simulink model "MAXWELL_Simulink"  (R2023a)
settings: Solver=FixedStepAuto  StartTime=0.0  StopTime=3600*4  FixedStep=5  MaxStep=10  RelTol=1e-7  AbsTol=1e-7
model workspace (MAT data in the model file):
  Gs = [0  0  0.707106781187  -0.707106781187; 0.707106781187  0.707106781187  -0.707106781187  -0.707106781187; 0.707106781187  -0.707106781187  0  0]
  Iws = 0.002
  OmegaRW_0 = [5000; 5000; 5000; 5000]
  Omega_bias = 26.1799
  RW_bias = 52.3598775598
undefined symbols (not defined in the file or in its folder): DiscIntNeverNeededParam, rad, s
libraries: slpidlib x3, dspinverses x3, sharedtransform x3, aerolibconvert2 x1, aerolibsatdyn x1, dspmathops x1, aerolibutil x1
settings Model: Creator=The MathWorks, Inc.  LastModifiedBy=TheBa
settings SolverCC: MaxConsecutiveMinStep=10  AutoInsertRateTranBlk=on  DecoupledContinuousIntegration=on  MinimalZcImpactIntegration=on  MaxZcPerStep=1
settings OptimizationCC: DefaultParameterBehavior=Inlined  UseDivisionForNetSlopeComputation=on  GainParamInheritBuiltInType=on  UseFloatMulNetSlope=on  InlineInvariantSignals=on  EfficientFloat2IntCast=on  LifeSpan=1
settings DebuggingCC: ReadBeforeWriteMsg=DisableAll  WriteAfterWriteMsg=DisableAll  WriteAfterReadMsg=DisableAll  MultiTaskDSMMsg=none  UnconnectedInputMsg=warning  UnconnectedOutputMsg=warning  UnconnectedLineMsg=warning
settings HardwareCC: ProdLongLongMode=on
settings ModelReferenceCC: UpdateModelReferenceTargets=IfOutOfDate  EnableRefExpFcnMdlSchedulingChecks=on
settings SFSimCC: SFSimEcho=off  MATLABDynamicMemAlloc=off
settings RTWCC: GenerateReport=on  BuildConfiguration=Faster Runs  LaunchReport=on  DLArmComputeVersion=19.05
settings CodeAppCC: ForceParamTrailComments=on
settings GRTTargetCC: CombineSignalStateStructs=on  MatFileLogging=off  SupportNonFinite=off  SupportVariableSizeSignals=on

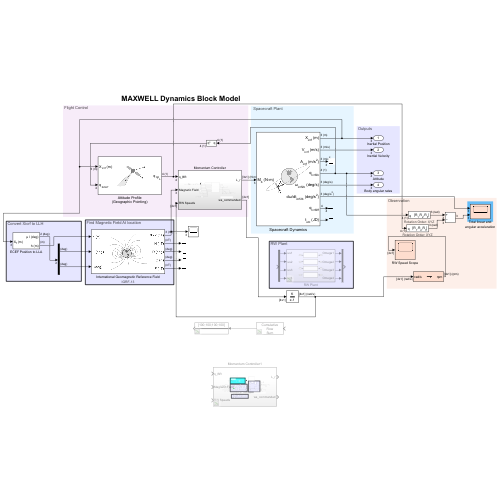
[thumbnail: Simulink's stored preview of the top-level diagram]
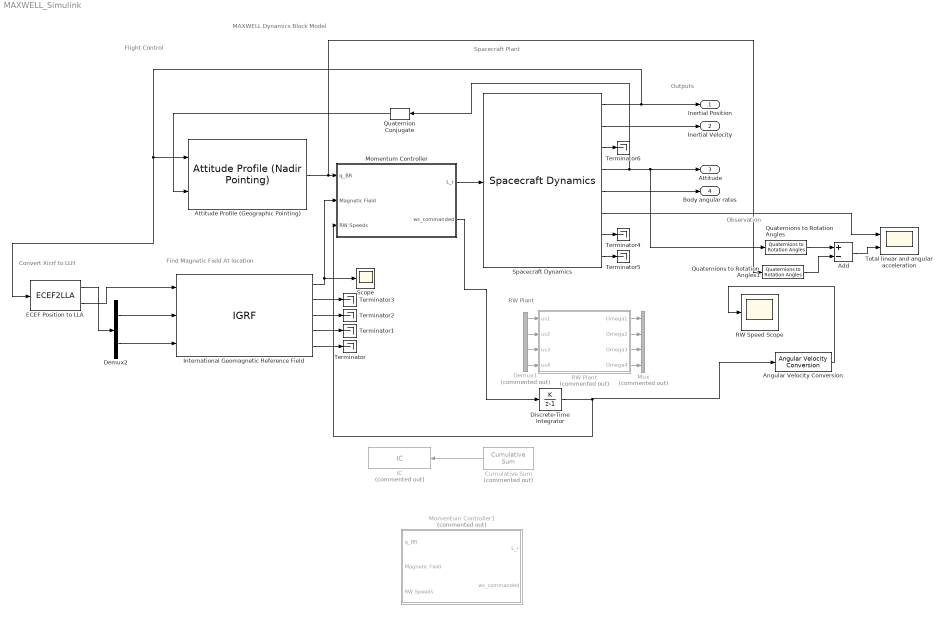
== system MAXWELL_Simulink ==
  note: RW Plant
  note: Convert Xicrf to LLH
  note: Flight Control
  note: Outputs
  note: Spacecraft Plant
  note: Observation
  note: MAXWELL Dynamics Block Model
  note: Find Magnetic Field At location
  Add : Sum  Inputs=+-
  Angular Velocity Conversion : aerolibconvert2/Angular Velocity Conversion  IU=rad/s  OU=rpm
  Attitude Profile (Geographic Pointing) : aerolibsatdyn/Attitude Profile (Nadir Pointing)  outputError=on  outputFinalAttitude=off  portFrame=ICRF  pointingMode=Point at nadir  celestialTarget=Sun  tunablePointing=off  primaryAlignmentSrc=Dialog  primaryAlignment=[0 0 1]  secondaryAlignmentSrc=Dialog  secondaryAlignment=[1 0 0]  constraintFrame=ICRF  primaryConstraintSrc=Dialog  primaryConstraint=[1 0 0]  secondaryConstraintSrc=Dialog  secondaryConstraint=[0 1 0]
      settings: LibrarySourceBlock=|
      | aerolibsatdyn/Attitude Profile
      | (Geographic Pointing)
  Cumulative Sum : dspmathops/Cumulative Sum  Commented=on  dim=Rows  reset_popup=None  roundingMode=Floor  overflowMode=off  outputDataTypeStr=Inherit: Same as accumulator  outputMin=[]  outputMax=[]  outputLastDataTypeStr=Inherit: Same as accumulator
  Demux1 : Demux  Commented=on
  Demux2 : Demux  Outputs=2
  Discrete-Time Integrator : DiscreteIntegrator  IntegratorMethod=Accumulation: Forward Euler  InitialCondition=[100;100;100;100]  SampleTime=-1  ICPrevOutput=DiscIntNeverNeededParam  ICPrevScaledInput=DiscIntNeverNeededParam
  ECEF Position to LLA : ECEF2LLA
  IC : InitialCondition  Commented=on  Value=[100;100;100;100]
  International Geomagnetic Reference Field : IGRF  time_in=off  month=January  day=1  year=2020  sv_out=off
      settings: AttributesFormatString=%<generation>
  Momentum Controller : Subsystem
  Momentum Controller1 : Subsystem  Commented=on
  Mux : Mux  Commented=on
  Quaternion Conjugate : aerolibutil/Quaternion Conjugate
  Quaternions to Rotation Angles : sharedtransform/Quaternions to Rotation Angles  rotationOrder=XYZ  aMode=aMode
  Quaternions to Rotation Angles1 : sharedtransform/Quaternions to Rotation Angles  rotationOrder=XYZ  aMode=aMode
  RW Plant : Subsystem  Commented=on
  RW Speed Scope : Scope
  Scope : Scope
  Spacecraft Dynamics : SpacecraftDynamics  forcesIn=off  outputAccel=on  startDate=2459216  mass=6  inertia=diag([10.5 8 6.75])  semiMajorAxis=6778140  eccentricity=0  inclination=20  raan=60  argPeriapsis=0  trueAnomaly=0  attitude=[0.0050 -0.5025 0.5025 -0.7035]  attitudeRate=[5 8 8]  outputAngAccel=on  outputTransform=on
  Terminator{,1..6} (7 alike) : Terminator
  Total linear and angular acceleration : Scope  NumInputPorts=2
  Inertial Position : Outport
  Inertial Velocity : Outport  Port=2
  Attitude : Outport  Port=3
  Body angular rates : Outport  Port=4
  wires:
  Spacecraft Dynamics/1 -> Inertial Position/1, Attitude Profile (Geographic Pointing)/1, ECEF Position to LLA/1
  Spacecraft Dynamics/4 -> Attitude/1, Quaternions to Rotation Angles/1, Quaternion Conjugate/1
  Quaternion Conjugate/1 -> Attitude Profile (Geographic Pointing)/2
  Spacecraft Dynamics/5 -> Body angular rates/1
  Demux1/1 -> RW Plant/1(us1)
  RW Plant/3(Omega3) -> Mux/3
  Demux1/3 -> RW Plant/3(us3)
  RW Plant/1(Omega1) -> Mux/1
  Demux1/4 -> RW Plant/4(us4)
  Demux1/2 -> RW Plant/2(us2)
  RW Plant/4(Omega4) -> Mux/4
  RW Plant/2(Omega2) -> Mux/2
  ECEF Position to LLA/2 -> International Geomagnetic Reference Field/1
  ECEF Position to LLA/1 -> Demux2/1
  Demux2/1 -> International Geomagnetic Reference Field/2
  Demux2/2 -> International Geomagnetic Reference Field/3
  International Geomagnetic Reference Field/1 -> Scope/1, Momentum Controller/2(Magnetic Field)
  Momentum Controller/1(L_r) -> Spacecraft Dynamics/1
  International Geomagnetic Reference Field/5 -> Terminator/1
  International Geomagnetic Reference Field/4 -> Terminator1/1
  International Geomagnetic Reference Field/3 -> Terminator2/1
  International Geomagnetic Reference Field/2 -> Terminator3/1
  Spacecraft Dynamics/7 -> Terminator4/1
  Spacecraft Dynamics/2 -> Inertial Velocity/1
  Attitude Profile (Geographic Pointing)/1 -> Quaternions to Rotation Angles1/1, Momentum Controller/1(q_BR)
  Spacecraft Dynamics/6 -> Total linear and angular acceleration/1
  Angular Velocity Conversion/1 -> RW Speed Scope/1
  Spacecraft Dynamics/3 -> Terminator6/1
  Spacecraft Dynamics/8 -> Terminator5/1
  Cumulative Sum/1 -> IC/1
  Momentum Controller/2(ws_commanded) -> Discrete-Time Integrator/1
  Discrete-Time Integrator/1 -> Momentum Controller/3(RW Speeds), Angular Velocity Conversion/1
  Quaternions to Rotation Angles/1 -> Add/1
  Add/1 -> Total linear and angular acceleration/2
  Quaternions to Rotation Angles1/1 -> Add/2

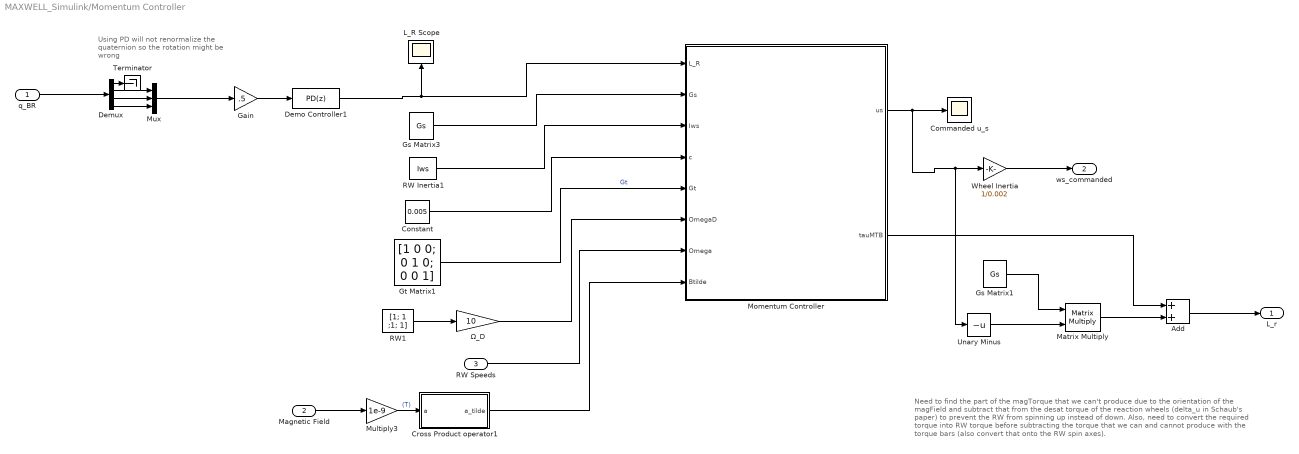
== system MAXWELL_Simulink/Momentum Controller ==
  note: Need to find the part of the magTorque that we can't produce due to the orientation of the magField and subtract that from the desat torque of the reaction wheels (delta_u in Schaub's paper) to prevent the RW from spinning up instead of down. Also, need to convert the required torque into RW torque before subtracting the torque that we can and cannot produce with the torque bars (also convert that onto the RW spin axes).
  note: Using PD will not renormalize the quaternion so the rotation might be wrong
  q_BR : Inport
  Magnetic Field : Inport  Port=2
  RW Speeds : Inport  Port=3
  Add : Sum
  "Commanded u_s " : Scope
  Constant : Constant  Value=0.005
  Cross Product operator1 : MATLAB Function  TreatAsAtomicUnit=on
  Demo Controller1 : slpidlib/PID Controller  Controller=PD  Form=Parallel  TimeDomain=Discrete-time  UseExternalTs=off  SampleTime=-1  IntegratorMethod=Trapezoidal  FilterMethod=Trapezoidal  ControllerParametersSource=internal  P=.0055  I=0  UseKiTs=off  D=.17  N=1  UseFilter=off  TunerSelectOption=Transfer Function Based (PID Tuner App)  InitialConditionSource=internal  InitialConditionForIntegrator=0  InitialConditionForFilter=0  DifferentiatorICPrevScaledInput=0  ExternalReset=none  TrackingMode=off  Kt=1  LimitOutput=on  SatLimitsSource=internal  UpperSaturationLimit=0.008  LowerSaturationLimit=-0.008  LinearizeAsGain=on  AntiWindupMode=none  Kb=1  LimitIntegrator=off  UpperIntegratorSaturationLimit=inf  LowerIntegratorSaturationLimit=-inf  POutMin=[]  POutMax=[]  IOutMin=[]  IOutMax=[]  DOutMin=[]  DOutMax=[]  NOutMin=[]  NOutMax=[]  SumOutMin=[]  SumOutMax=[]  SaturationOutMin=[]  SaturationOutMax=[]  PParamMin=[]  PParamMax=[]  IParamMin=[]  IParamMax=[]  DParamMin=[]  DParamMax=[]  NParamMin=[]  NParamMax=[]  KbParamMin=[]  KbParamMax=[]  KtParamMin=[]  KtParamMax=[]  KbOutMin=[]  KbOutMax=[]  KtOutMin=[]  KtOutMax=[]  IntegratorOutMin=[]  IntegratorOutMax=[]  FilterOutMin=[]  FilterOutMax=[]  SumI1OutMin=[]  SumI1OutMax=[]  SumI2OutMin=[]  SumI2OutMax=[]  SumI3OutMin=[]  SumI3OutMax=[]  SumI4OutMin=[]  SumI4OutMax=[]  SumDOutMin=[]  SumDOutMax=[]  DifferentiatorOutMin=[]  DifferentiatorOutMax=[]  FilterDiffOutCoefMin=[]  FilterDiffOutCoefMax=[]  ReciprocalOutMin=[]  ReciprocalOutMax=[]  SumDenOutMin=[]  SumDenOutMax=[]  SumNumOutMin=[]  SumNumOutMax=[]  DivideOutMin=[]  DivideOutMax=[]  UdiffTsProdOutMin=[]  UdiffTsProdOutMax=[]  NTsProdOutMin=[]  NTsProdOutMax=[]  UintegralTsProdOutMin=[]  UintegralTsProdOutMax=[]  UngainTsProdOutMin=[]  UngainTsProdOutMax=[]  ClampingZeroOutDataTypeStr=Inherit: Inherit via back propagation  ClampingZeroOutMin=[]  ClampingZeroOutMax=[]  FilterDenConstantOutDataTypeStr=Inherit: Inherit via back propagation  FilterDenConstantOutMin=[]  FilterDenConstantOutMax=[]  PCopyOutDataTypeStr=Inherit: Inherit via back propagation  PCopyOutMin=[]  PCopyOutMax=[]  NCopyOutDataTypeStr=Inherit: Inherit via back propagation  NCopyOutMin=[]  NCopyOutMax=[]  IntegratorContinuousStateAttributes=''  IntegratorStateMustResolveToSignalObject=off  IntegratorRTWStateStorageClass=Auto  FilterContinuousStateAttributes=''  FilterStateMustResolveToSignalObject=off  FilterRTWStateStorageClass=Auto  ParallelPVariant=InternalParameters  IdealPVariant=Disabled  IVariant=Disabled  DVariant=InternalParameters  IntegratorVariant=Disabled  SatVariant=Enabled  AWVariant=Disabled  PCopyVariant=Disabled  TRVariant=Disabled  FdbkBlocksVariant=Forward  IdealPFdbkVariant=Disabled  SatFdbkVariant=Disabled  DerivativeFilterVariant=Differentiator  NVariant=Passthrough  NCopyVariant=Disabled_SignalSpec  FilterICVariant=InternalICsDifferentiator  IntegratorICVariant=Disabled  ExternalResetVariant=Disabled  TRSumVariant=Passthrough  SumFdbkVariant=Disabled  SumVariant=Sum_PD  TsampFilterVariant=InternalTs  TsampNgainVariant=Passthrough  TsampIntegralVariant=Disabled_SignalSpec  ExternalSaturationOutDataTypeStr=Inherit: Same as second input
  Demux : Demux
  Gain : Gain  Gain=.5
  Gs Matrix1 : Constant  Value=Gs
  Gs Matrix3 : Constant  Value=Gs
  Gt Matrix1 : Constant  Value=[1 0 0; 0 1 0; 0 0 1]
  L_R Scope : Scope
  Matrix Multiply : Product  Multiplication=Matrix(*)
  Momentum Controller : MATLAB Function  TreatAsAtomicUnit=on
  Multiply3 : Gain  Gain=1e-9
  Mux : Mux  Inputs=3
  RW Inertia1 : Constant  Value=Iws
  RW1 : Constant  Value=[1; 1 ;1; 1]
  Terminator : Terminator
  Unary Minus : UnaryMinus
  Wheel Inertia : Gain  Gain=1/0.002
  Ω_D : Gain  Gain=10
  L_r : Outport
  ws_commanded : Outport  Port=2
  wires:
  Multiply3/1 -> Cross Product operator1/1(a)  "(T)"
  RW1/1 -> Ω_D/1
  Magnetic Field/1 -> Multiply3/1
  Wheel Inertia/1 -> ws_commanded/1
  Demux/2 -> Mux/1
  Demux/3 -> Mux/2
  Demux/4 -> Mux/3
  Demux/1 -> Terminator/1
  Mux/1 -> Gain/1
  Gain/1 -> Demo Controller1/1
  q_BR/1 -> Demux/1
  Demo Controller1/1 -> Momentum Controller/1(L_R), L_R Scope/1
  Gs Matrix3/1 -> Momentum Controller/2(Gs)
  RW Inertia1/1 -> Momentum Controller/3(Iws)
  Constant/1 -> Momentum Controller/4(c)
  Ω_D/1 -> Momentum Controller/6(OmegaD)
  Gt Matrix1/1 -> Momentum Controller/5(Gt)  "Gt"
  RW Speeds/1 -> Momentum Controller/7(Omega)
  Cross Product operator1/1(a_tilde) -> Momentum Controller/8(Btilde)
  Momentum Controller/1(us) -> Unary Minus/1, Wheel Inertia/1, "Commanded u_s "/1
  Gs Matrix1/1 -> Matrix Multiply/1
  Unary Minus/1 -> Matrix Multiply/2
  Matrix Multiply/1 -> Add/2
  Add/1 -> L_r/1
  Momentum Controller/2(tauMTB) -> Add/1

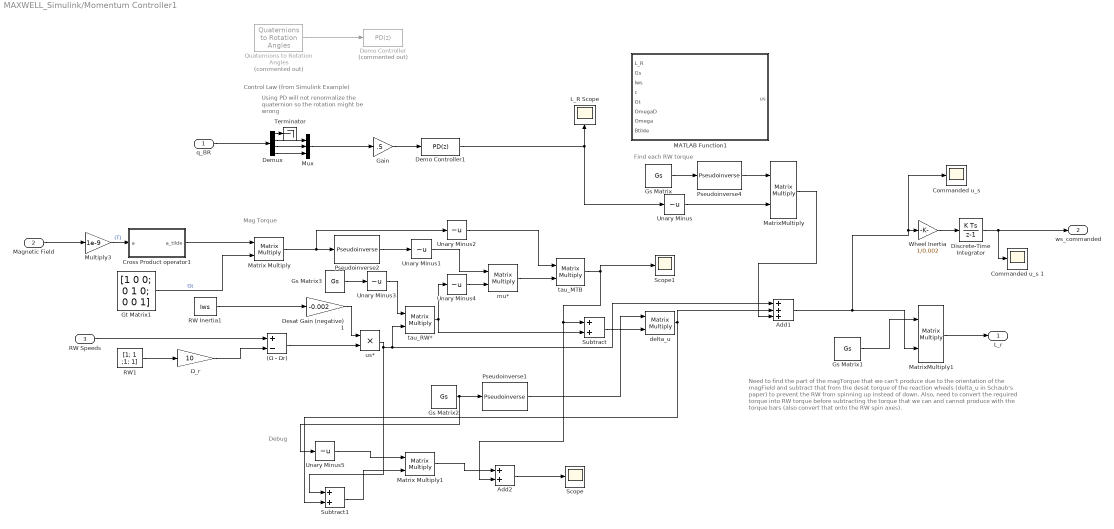
== system MAXWELL_Simulink/Momentum Controller1 ==
  note: Need to find the part of the magTorque that we can't produce due to the orientation of the magField and subtract that from the desat torque of the reaction wheels (delta_u in Schaub's paper) to prevent the RW from spinning up instead of down. Also, need to convert the required torque into RW torque before subtracting the torque that we can and cannot produce with the torque bars (also convert that onto the RW spin axes).
  note: Control Law (from Simulink Example)
  note: Mag Torque
  note: Find each RW torque
  note: Using PD will not renormalize the quaternion so the rotation might be wrong
  note: Debug
  q_BR : Inport
  Magnetic Field : Inport  Port=2
  RW Speeds : Inport  Port=3
  (Ω - Ωr) : Sum  Inputs=+-
  Add1 : Sum  Inputs=+++
  Add2 : Sum
  "Commanded u_s " : Scope
  Commanded u_s 1 : Scope
  Cross Product operator1 : MATLAB Function  TreatAsAtomicUnit=on
  Demo Controller : slpidlib/PID Controller  Commented=on  Controller=PD  Form=Parallel  TimeDomain=Discrete-time  UseExternalTs=off  SampleTime=-1  IntegratorMethod=Trapezoidal  FilterMethod=Trapezoidal  ControllerParametersSource=internal  P=.000055  I=0  UseKiTs=off  D=.017  N=1  UseFilter=off  TunerSelectOption=Transfer Function Based (PID Tuner App)  InitialConditionSource=internal  InitialConditionForIntegrator=0  InitialConditionForFilter=0  DifferentiatorICPrevScaledInput=0  ExternalReset=none  TrackingMode=off  Kt=1  LimitOutput=on  SatLimitsSource=internal  UpperSaturationLimit=0.008  LowerSaturationLimit=-0.008  LinearizeAsGain=on  AntiWindupMode=none  Kb=1  LimitIntegrator=off  UpperIntegratorSaturationLimit=inf  LowerIntegratorSaturationLimit=-inf  POutMin=[]  POutMax=[]  IOutMin=[]  IOutMax=[]  DOutMin=[]  DOutMax=[]  NOutMin=[]  NOutMax=[]  SumOutMin=[]  SumOutMax=[]  SaturationOutMin=[]  SaturationOutMax=[]  PParamMin=[]  PParamMax=[]  IParamMin=[]  IParamMax=[]  DParamMin=[]  DParamMax=[]  NParamMin=[]  NParamMax=[]  KbParamMin=[]  KbParamMax=[]  KtParamMin=[]  KtParamMax=[]  KbOutMin=[]  KbOutMax=[]  KtOutMin=[]  KtOutMax=[]  IntegratorOutMin=[]  IntegratorOutMax=[]  FilterOutMin=[]  FilterOutMax=[]  SumI1OutMin=[]  SumI1OutMax=[]  SumI2OutMin=[]  SumI2OutMax=[]  SumI3OutMin=[]  SumI3OutMax=[]  SumI4OutMin=[]  SumI4OutMax=[]  SumDOutMin=[]  SumDOutMax=[]  DifferentiatorOutMin=[]  DifferentiatorOutMax=[]  FilterDiffOutCoefMin=[]  FilterDiffOutCoefMax=[]  ReciprocalOutMin=[]  ReciprocalOutMax=[]  SumDenOutMin=[]  SumDenOutMax=[]  SumNumOutMin=[]  SumNumOutMax=[]  DivideOutMin=[]  DivideOutMax=[]  UdiffTsProdOutMin=[]  UdiffTsProdOutMax=[]  NTsProdOutMin=[]  NTsProdOutMax=[]  UintegralTsProdOutMin=[]  UintegralTsProdOutMax=[]  UngainTsProdOutMin=[]  UngainTsProdOutMax=[]  ClampingZeroOutDataTypeStr=Inherit: Inherit via back propagation  ClampingZeroOutMin=[]  ClampingZeroOutMax=[]  FilterDenConstantOutDataTypeStr=Inherit: Inherit via back propagation  FilterDenConstantOutMin=[]  FilterDenConstantOutMax=[]  PCopyOutDataTypeStr=Inherit: Inherit via back propagation  PCopyOutMin=[]  PCopyOutMax=[]  NCopyOutDataTypeStr=Inherit: Inherit via back propagation  NCopyOutMin=[]  NCopyOutMax=[]  IntegratorContinuousStateAttributes=''  IntegratorStateMustResolveToSignalObject=off  IntegratorRTWStateStorageClass=Auto  FilterContinuousStateAttributes=''  FilterStateMustResolveToSignalObject=off  FilterRTWStateStorageClass=Auto  ParallelPVariant=InternalParameters  IdealPVariant=Disabled  IVariant=Disabled  DVariant=InternalParameters  IntegratorVariant=Disabled  SatVariant=Enabled  AWVariant=Disabled  PCopyVariant=Disabled  TRVariant=Disabled  FdbkBlocksVariant=Forward  IdealPFdbkVariant=Disabled  SatFdbkVariant=Disabled  DerivativeFilterVariant=Differentiator  NVariant=Passthrough  NCopyVariant=Disabled_SignalSpec  FilterICVariant=InternalICsDifferentiator  IntegratorICVariant=Disabled  ExternalResetVariant=Disabled  TRSumVariant=Passthrough  SumFdbkVariant=Disabled  SumVariant=Sum_PD  TsampFilterVariant=InternalTs  TsampNgainVariant=Passthrough  TsampIntegralVariant=Disabled_SignalSpec  ExternalSaturationOutDataTypeStr=Inherit: Same as second input
  Demo Controller1 : slpidlib/PID Controller  Controller=PD  Form=Parallel  TimeDomain=Discrete-time  UseExternalTs=off  SampleTime=-1  IntegratorMethod=Trapezoidal  FilterMethod=Trapezoidal  ControllerParametersSource=internal  P=.0055  I=0  UseKiTs=off  D=.17  N=1  UseFilter=off  TunerSelectOption=Transfer Function Based (PID Tuner App)  InitialConditionSource=internal  InitialConditionForIntegrator=0  InitialConditionForFilter=0  DifferentiatorICPrevScaledInput=0  ExternalReset=none  TrackingMode=off  Kt=1  LimitOutput=on  SatLimitsSource=internal  UpperSaturationLimit=0.008  LowerSaturationLimit=-0.008  LinearizeAsGain=on  AntiWindupMode=none  Kb=1  LimitIntegrator=off  UpperIntegratorSaturationLimit=inf  LowerIntegratorSaturationLimit=-inf  POutMin=[]  POutMax=[]  IOutMin=[]  IOutMax=[]  DOutMin=[]  DOutMax=[]  NOutMin=[]  NOutMax=[]  SumOutMin=[]  SumOutMax=[]  SaturationOutMin=[]  SaturationOutMax=[]  PParamMin=[]  PParamMax=[]  IParamMin=[]  IParamMax=[]  DParamMin=[]  DParamMax=[]  NParamMin=[]  NParamMax=[]  KbParamMin=[]  KbParamMax=[]  KtParamMin=[]  KtParamMax=[]  KbOutMin=[]  KbOutMax=[]  KtOutMin=[]  KtOutMax=[]  IntegratorOutMin=[]  IntegratorOutMax=[]  FilterOutMin=[]  FilterOutMax=[]  SumI1OutMin=[]  SumI1OutMax=[]  SumI2OutMin=[]  SumI2OutMax=[]  SumI3OutMin=[]  SumI3OutMax=[]  SumI4OutMin=[]  SumI4OutMax=[]  SumDOutMin=[]  SumDOutMax=[]  DifferentiatorOutMin=[]  DifferentiatorOutMax=[]  FilterDiffOutCoefMin=[]  FilterDiffOutCoefMax=[]  ReciprocalOutMin=[]  ReciprocalOutMax=[]  SumDenOutMin=[]  SumDenOutMax=[]  SumNumOutMin=[]  SumNumOutMax=[]  DivideOutMin=[]  DivideOutMax=[]  UdiffTsProdOutMin=[]  UdiffTsProdOutMax=[]  NTsProdOutMin=[]  NTsProdOutMax=[]  UintegralTsProdOutMin=[]  UintegralTsProdOutMax=[]  UngainTsProdOutMin=[]  UngainTsProdOutMax=[]  ClampingZeroOutDataTypeStr=Inherit: Inherit via back propagation  ClampingZeroOutMin=[]  ClampingZeroOutMax=[]  FilterDenConstantOutDataTypeStr=Inherit: Inherit via back propagation  FilterDenConstantOutMin=[]  FilterDenConstantOutMax=[]  PCopyOutDataTypeStr=Inherit: Inherit via back propagation  PCopyOutMin=[]  PCopyOutMax=[]  NCopyOutDataTypeStr=Inherit: Inherit via back propagation  NCopyOutMin=[]  NCopyOutMax=[]  IntegratorContinuousStateAttributes=''  IntegratorStateMustResolveToSignalObject=off  IntegratorRTWStateStorageClass=Auto  FilterContinuousStateAttributes=''  FilterStateMustResolveToSignalObject=off  FilterRTWStateStorageClass=Auto  ParallelPVariant=InternalParameters  IdealPVariant=Disabled  IVariant=Disabled  DVariant=InternalParameters  IntegratorVariant=Disabled  SatVariant=Enabled  AWVariant=Disabled  PCopyVariant=Disabled  TRVariant=Disabled  FdbkBlocksVariant=Forward  IdealPFdbkVariant=Disabled  SatFdbkVariant=Disabled  DerivativeFilterVariant=Differentiator  NVariant=Passthrough  NCopyVariant=Disabled_SignalSpec  FilterICVariant=InternalICsDifferentiator  IntegratorICVariant=Disabled  ExternalResetVariant=Disabled  TRSumVariant=Passthrough  SumFdbkVariant=Disabled  SumVariant=Sum_PD  TsampFilterVariant=InternalTs  TsampNgainVariant=Passthrough  TsampIntegralVariant=Disabled_SignalSpec  ExternalSaturationOutDataTypeStr=Inherit: Same as second input
  Demux : Demux
  Desat Gain (negative) 1 : Gain  Gain=-0.002
  Discrete-Time Integrator : DiscreteIntegrator  SampleTime=-1  ICPrevOutput=DiscIntNeverNeededParam  ICPrevScaledInput=DiscIntNeverNeededParam
  Gain : Gain  Gain=.5
  Gs Matrix{,1..3} (4 alike) : Constant  Value=Gs
  Gt Matrix1 : Constant  Value=[1 0 0; 0 1 0; 0 0 1]
  L_R Scope : Scope
  MATLAB Function1 : MATLAB Function  TreatAsAtomicUnit=on
  Matrix Multiply : Product  Multiplication=Matrix(*)
  Matrix Multiply1 : Product  Multiplication=Matrix(*)
  MatrixMultiply : Product  Multiplication=Matrix(*)
  MatrixMultiply1 : Product  Multiplication=Matrix(*)
  Multiply3 : Gain  Gain=1e-9
  Mux : Mux  Inputs=3
  Pseudoinverse1 : dspinverses/Pseudoinverse  wanterr=off  SimulateUsing=Interpreted execution
  Pseudoinverse2 : dspinverses/Pseudoinverse  wanterr=off  SimulateUsing=Interpreted execution
  Pseudoinverse4 : dspinverses/Pseudoinverse  wanterr=off  SimulateUsing=Interpreted execution
  Quaternions to Rotation Angles : sharedtransform/Quaternions to Rotation Angles  Commented=on  rotationOrder=XYZ  aMode=aMode
  RW Inertia1 : Constant  Value=Iws
  RW1 : Constant  Value=[1; 1 ;1; 1]
  Scope : Scope
  Scope1 : Scope
  Subtract : Sum
  Subtract1 : Sum
  Terminator : Terminator
  Unary Minus{,1..5} (6 alike) : UnaryMinus
  Wheel Inertia : Gain  Gain=1/0.002
  delta_u : Product  Multiplication=Matrix(*)
  mu* : Product  Multiplication=Matrix(*)
  tau_MTB : Product  Multiplication=Matrix(*)
  tau_RW* : Product  Multiplication=Matrix(*)
  us* : Product
  Ω_r : Gain  Gain=10
  L_r : Outport
  ws_commanded : Outport  Port=2
  wires:
  Quaternions to Rotation Angles/1 -> Demo Controller/1
  Gs Matrix/1 -> Pseudoinverse4/1
  Multiply3/1 -> Cross Product operator1/1(a)  "(T)"
  RW1/1 -> Ω_r/1
  Ω_r/1 -> (Ω - Ωr)/2
  RW Speeds/1 -> (Ω - Ωr)/1
  Magnetic Field/1 -> Multiply3/1
  RW Inertia1/1 -> Desat Gain (negative) 1/1
  (Ω - Ωr)/1 -> us*/2
  Desat Gain (negative) 1/1 -> us*/1
  us*/1 -> Subtract1/1, Add1/1, tau_RW*/2
  Gs Matrix3/1 -> Unary Minus3/1
  Matrix Multiply/1 -> Unary Minus2/1, Pseudoinverse2/1
  Pseudoinverse2/1 -> Unary Minus1/1
  Unary Minus1/1 -> mu*/1
  mu*/1 -> tau_MTB/2
  Unary Minus2/1 -> tau_MTB/1
  Pseudoinverse4/1 -> MatrixMultiply/1
  Wheel Inertia/1 -> Discrete-Time Integrator/1
  Discrete-Time Integrator/1 -> Commanded u_s 1/1, ws_commanded/1
  Demux/2 -> Mux/1
  Demux/3 -> Mux/2
  Demux/4 -> Mux/3
  Demux/1 -> Terminator/1
  Mux/1 -> Gain/1
  Gain/1 -> Demo Controller1/1
  q_BR/1 -> Demux/1
  Demo Controller1/1 -> L_R Scope/1, Unary Minus/1
  tau_MTB/1 -> Scope1/1, Add2/2, Subtract/1
  Gs Matrix2/1 -> Unary Minus5/1, Pseudoinverse1/1
  Subtract/1 -> delta_u/2
  Pseudoinverse1/1 -> delta_u/1
  Unary Minus3/1 -> tau_RW*/1
  tau_RW*/1 -> Unary Minus4/1, Subtract/2
  Unary Minus4/1 -> mu*/2
  Unary Minus/1 -> MatrixMultiply/2
  delta_u/1 -> Subtract1/2, Add1/2
  Add1/1 -> MatrixMultiply1/2, "Commanded u_s "/1, Wheel Inertia/1
  MatrixMultiply/1 -> Add1/3
  Cross Product operator1/1(a_tilde) -> Matrix Multiply/1
  Gt Matrix1/1 -> Matrix Multiply/2  "Gt"
  Unary Minus5/1 -> Matrix Multiply1/1
  Subtract1/1 -> Matrix Multiply1/2
  Matrix Multiply1/1 -> Add2/1
  Add2/1 -> Scope/1
  Gs Matrix1/1 -> MatrixMultiply1/1
  MatrixMultiply1/1 -> L_r/1

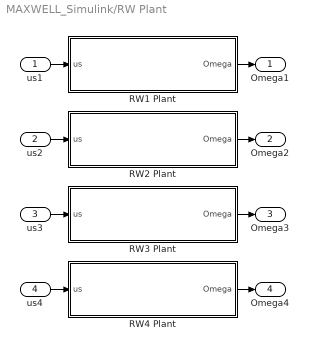
== system MAXWELL_Simulink/RW Plant ==
  us1 : Inport
  us2 : Inport  Port=2
  us3 : Inport  Port=3
  us4 : Inport  Port=4
  RW1 Plant : Subsystem
  RW2 Plant : Subsystem
  RW3 Plant : Subsystem
  RW4 Plant : Subsystem
  Omega1 : Outport
  Omega2 : Outport  Port=2
  Omega3 : Outport  Port=3
  Omega4 : Outport  Port=4
  wires:
  RW1 Plant/1(Omega) -> Omega1/1
  us3/1 -> RW3 Plant/1(us)
  us4/1 -> RW4 Plant/1(us)
  us2/1 -> RW2 Plant/1(us)
  RW3 Plant/1(Omega) -> Omega3/1
  RW2 Plant/1(Omega) -> Omega2/1
  RW4 Plant/1(Omega) -> Omega4/1
  us1/1 -> RW1 Plant/1(us)

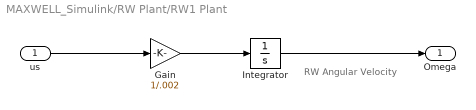
== system MAXWELL_Simulink/RW Plant/RW1 Plant ==
  note: RW Angular Velocity
  us : Inport
  Gain : Gain  Gain=1/.002
  Integrator : Integrator
  Omega : Outport
  wires:
  us/1 -> Gain/1
  Integrator/1 -> Omega/1
  Gain/1 -> Integrator/1

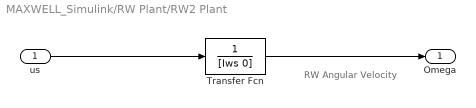
== system MAXWELL_Simulink/RW Plant/RW2 Plant ==
  note: RW Angular Velocity
  us : Inport
  Transfer Fcn : TransferFcn  Denominator=[Iws 0]
  Omega : Outport
  wires:
  us/1 -> Transfer Fcn/1
  Transfer Fcn/1 -> Omega/1

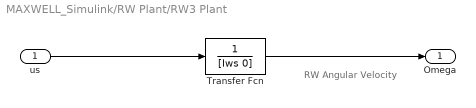
== system MAXWELL_Simulink/RW Plant/RW3 Plant ==
  note: RW Angular Velocity
  us : Inport
  Transfer Fcn : TransferFcn  Denominator=[Iws 0]
  Omega : Outport
  wires:
  us/1 -> Transfer Fcn/1
  Transfer Fcn/1 -> Omega/1

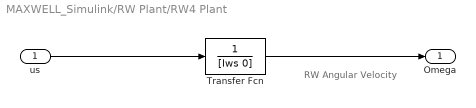
== system MAXWELL_Simulink/RW Plant/RW4 Plant ==
  note: RW Angular Velocity
  us : Inport
  Transfer Fcn : TransferFcn  Denominator=[Iws 0]
  Omega : Outport
  wires:
  us/1 -> Transfer Fcn/1
  Transfer Fcn/1 -> Omega/1

== matlab function MAXWELL_Simulink/Momentum Controller/Cross Product operator1 ==
  data: a input; a_tilde output
function a_tilde  = tilde(a)
%tilde(a) Returns the tilde matrix of the vector 'a' (3 dim)

% Throw error if vector has more than 3 elements
if numel(a) > 3
    error('Your vector is too long')
end

% Decompose vector into elements
a1 = a(1); a2 = a(2); a3 = a(3);

% Construct tilde matrix
a_tilde = [ 0 -a3 a2; a3 0 -a1; -a2 a1 0];
end

== matlab function MAXWELL_Simulink/Momentum Controller/Momentum Controller ==
  data: L_R input; us output; Gs input; Iws input; c input; Gt input; OmegaD input; Omega input; Btilde input; tauMTB output
function [us,tauMTB] = WheelTorque_Command(L_R, Gs, Iws, c, Gt, OmegaD, Omega, Btilde )       %remove error? 

    % Find required RW torque to point
    usReq = pinv(Gs) * (- L_R); % [Nm]

    % Find despin torque
    usStar = -c * Iws * (Omega - OmegaD); % [Nm] ---

    % Find required magnetic dipole
    muStar = -pinv(Btilde*Gt) * Gs * usStar;   %---

    % Find resulitng magnetic torque
    tauMTB = -Btilde * Gt * muStar; % [Nm]        %---

    % Find the component of torque that cannot be produced by the MTB
    deltaU = pinv(Gs) * (tauMTB - Gs * usStar); % [Nm]    ---

    % Find actual applied RW torque (don't make it try despin if MTB cannot
    % produce counter torque in that direction)
    us = usReq + usStar + deltaU; % [Nm]
    % us = usReq;

== matlab function MAXWELL_Simulink/Momentum Controller1/Cross Product operator1 ==
  data: a input; a_tilde output
function a_tilde  = tilde(a)
%tilde(a) Returns the tilde matrix of the vector 'a' (3 dim)

% Throw error if vector has more than 3 elements
if numel(a) > 3
    error('Your vector is too long')
end

% Decompose vector into elements
a1 = a(1); a2 = a(2); a3 = a(3);

% Construct tilde matrix
a_tilde = [ 0 -a3 a2; a3 0 -a1; -a2 a1 0];
end

== matlab function MAXWELL_Simulink/Momentum Controller1/MATLAB Function1 ==
  data: L_R input; us output; Gs input; Iws input; c input; Gt input; OmegaD input; Omega input; Btilde input
function us = fcn(L_R, Gs, Iws, c, Gt, OmegaD, Omega, Btilde )       %remove error? 

    % Find required RW torque to point
    usReq = pinv(Gs) * (- L_R); % [Nm]

    % Find despin torque
    usStar = -c * Iws * (Omega - OmegaD); % [Nm] ---

    % Find required magnetic dipole
    muStar = -pinv(Btilde*Gt) * Gs * usStar;   %---

    % Find resulitng magnetic torque
    tauMTB = -Btilde * Gt * muStar; % [Nm]        %---

    % Find the component of torque that cannot be produced by the MTB
    deltaU = pinv(Gs) * (tauMTB - Gs * usStar); % [Nm]    ---

    % Find actual applied RW torque (don't make it try despin if MTB cannot
    % produce counter torque in that direction)
    us = usReq + usStar + deltaU; % [Nm]
